simulink model "maddenlibrary"  (R2012b)
settings: Solver=ode45  StartTime=0.0  StopTime=10.0  RelTol=1e-3
values from neighbouring files (symbols this model uses):
  T = 95/2    (= 47.5)    [fluxrampdemodsim.m]
undefined symbols (not defined in the file or in its folder): A, FRA, FRT, pfb_coeff_gen_calc, RS, T2, V
undefined symbols (not defined in the file): SL, transtable
libraries: xbsIndex_r4 x10038, casper_library_misc x83, casper_library_delays x22, xps_library x19, simulink x3, maddogLibrary x1
(part 13 of 106)

== system maddenlibrary/FRD/PhaseUnwrap ==
  note: FixPosJump
  note: Fix Neg Jup
  note: Determine If Phase Jump
  note: Calculate if we have Phase Jump
      | by comparing derivative of phase wrt time
      | to pi and -pi.
  note: Perform Phase Unwrap by adding
      | 0 , 2pi or -2pi
  note: State 0 : Add 0 to phase
      | Sate 1: Add 2pi to phase
      | State 2: Add -2pi to phase
      | State 3: Error
  note: Phase Unwrap
  note: State Machine Next State
  note: Error Flag Output
  note: Phase Addend:
      | 0.0, 2pi or -2pi
  note: Calc. Unwrapped
      | Phase
  note: How the muxes work
      |
      | always @(posedge clk)
      | //NextStae Mux
      | switch State:
      | {
      | 	0: //add 0 to phase
      | 		switch {negjmp, posjmp}
      | 		{
      | 			0: state<=0; break;
      | 			1: state,=1;break
      | 			2:state <=2; break
      | 			3:state <=3;
      | 		}
      | 		break
      |
      | 	1: // add
  Phase : Inport
  Rst : Inport  Port=2
  vld_in : Inport  Port=3
  mag_in : Inport  Port=4
  AddSub : xbsIndex_r4/AddSub  mode=Addition  use_carryin=off  use_carryout=off  en=off  latency=1  precision=User Defined  arith_type="Signed  (2's comp)"  n_bits=16  bin_pt=13  quantization=Truncate  overflow=Wrap  dbl_ovrd=off  use_behavioral_HDL=off  hw_selection=Fabric  pipelined=off  block_type=addsub
  Concat : xbsIndex_r4/Concat  num_inputs=2  dbl_ovrd=off  block_type=concat
  Constant : xbsIndex_r4/Constant  const=0  gui_display_data_type=Fixed-point  arith_type=Signed (2's comp)  n_bits=16  bin_pt=13  preci_type=Single  exp_width=8  frac_width=24  explicit_period=on  period=1  equ=P=C  opselect=C  inp2=PCIN>>17  opr=+  inp1=P  carry=CIN  dbl_ovrd=off  block_type=constant
  Constant1 : xbsIndex_r4/Constant  const=2  gui_display_data_type=Fixed-point  arith_type=Signed (2's comp)  n_bits=16  bin_pt=13  preci_type=Single  exp_width=8  frac_width=24  explicit_period=on  period=1  equ=P=C  opselect=C  inp2=PCIN>>17  opr=+  inp1=P  carry=CIN  dbl_ovrd=off  block_type=constant
  Constant10 : xbsIndex_r4/Constant  const=0  gui_display_data_type=Fixed-point  arith_type=Unsigned  n_bits=2  bin_pt=0  preci_type=Single  exp_width=8  frac_width=24  explicit_period=on  period=1  equ=P=C  opselect=C  inp2=PCIN>>17  opr=+  inp1=P  carry=CIN  dbl_ovrd=off  block_type=constant
  Constant{8,11..13,15,17} (6 alike) : xbsIndex_r4/Constant  const=3  gui_display_data_type=Fixed-point  arith_type=Unsigned  n_bits=2  bin_pt=0  preci_type=Single  exp_width=8  frac_width=24  explicit_period=on  period=1  equ=P=C  opselect=C  inp2=PCIN>>17  opr=+  inp1=P  carry=CIN  dbl_ovrd=off  block_type=constant
  Constant14 : xbsIndex_r4/Constant  const=0  gui_display_data_type=Fixed-point  arith_type=Unsigned  n_bits=2  bin_pt=0  preci_type=Single  exp_width=8  frac_width=24  explicit_period=on  period=1  equ=P=C  opselect=C  inp2=PCIN>>17  opr=+  inp1=P  carry=CIN  dbl_ovrd=off  block_type=constant
  Constant16 : xbsIndex_r4/Constant  const=2  gui_display_data_type=Fixed-point  arith_type=Unsigned  n_bits=2  bin_pt=0  preci_type=Single  exp_width=8  frac_width=24  explicit_period=on  period=1  equ=P=C  opselect=C  inp2=PCIN>>17  opr=+  inp1=P  carry=CIN  dbl_ovrd=off  block_type=constant
  Constant18 : xbsIndex_r4/Constant  const=0  gui_display_data_type=Boolean  arith_type=Boolean  n_bits=2  bin_pt=0  preci_type=Single  exp_width=8  frac_width=24  explicit_period=on  period=1  equ=P=C  opselect=C  inp2=PCIN>>17  opr=+  inp1=P  carry=CIN  dbl_ovrd=off  block_type=constant
  Constant19 : xbsIndex_r4/Constant  const=1  gui_display_data_type=Boolean  arith_type=Boolean  n_bits=2  bin_pt=0  preci_type=Single  exp_width=8  frac_width=24  explicit_period=on  period=1  equ=P=C  opselect=C  inp2=PCIN>>17  opr=+  inp1=P  carry=CIN  dbl_ovrd=off  block_type=constant
  Constant2 : xbsIndex_r4/Constant  const=-2  gui_display_data_type=Fixed-point  arith_type=Signed (2's comp)  n_bits=16  bin_pt=13  preci_type=Single  exp_width=8  frac_width=24  explicit_period=on  period=1  equ=P=C  opselect=C  inp2=PCIN>>17  opr=+  inp1=P  carry=CIN  dbl_ovrd=off  block_type=constant
  Constant3 : xbsIndex_r4/Constant  const=-1  gui_display_data_type=Fixed-point  arith_type=Signed (2's comp)  n_bits=16  bin_pt=13  preci_type=Single  exp_width=8  frac_width=24  explicit_period=on  period=1  equ=P=C  opselect=C  inp2=PCIN>>17  opr=+  inp1=P  carry=CIN  dbl_ovrd=off  block_type=constant
  Constant4 : xbsIndex_r4/Constant  const=1.0  gui_display_data_type=Fixed-point  arith_type=Signed (2's comp)  n_bits=16  bin_pt=13  preci_type=Single  exp_width=8  frac_width=24  explicit_period=on  period=1  equ=P=C  opselect=C  inp2=PCIN>>17  opr=+  inp1=P  carry=CIN  dbl_ovrd=off  block_type=constant
  Constant5 : xbsIndex_r4/Constant  const=0  gui_display_data_type=Fixed-point  arith_type=Unsigned  n_bits=2  bin_pt=0  preci_type=Single  exp_width=8  frac_width=24  explicit_period=on  period=1  equ=P=C  opselect=C  inp2=PCIN>>17  opr=+  inp1=P  carry=CIN  dbl_ovrd=off  block_type=constant
  Constant6 : xbsIndex_r4/Constant  const=2  gui_display_data_type=Fixed-point  arith_type=Unsigned  n_bits=2  bin_pt=0  preci_type=Single  exp_width=8  frac_width=24  explicit_period=on  period=1  equ=P=C  opselect=C  inp2=PCIN>>17  opr=+  inp1=P  carry=CIN  dbl_ovrd=off  block_type=constant
  Constant7 : xbsIndex_r4/Constant  const=1  gui_display_data_type=Fixed-point  arith_type=Unsigned  n_bits=2  bin_pt=0  preci_type=Single  exp_width=8  frac_width=24  explicit_period=on  period=1  equ=P=C  opselect=C  inp2=PCIN>>17  opr=+  inp1=P  carry=CIN  dbl_ovrd=off  block_type=constant
  Constant9 : xbsIndex_r4/Constant  const=1  gui_display_data_type=Fixed-point  arith_type=Unsigned  n_bits=2  bin_pt=0  preci_type=Single  exp_width=8  frac_width=24  explicit_period=on  period=1  equ=P=C  opselect=C  inp2=PCIN>>17  opr=+  inp1=P  carry=CIN  dbl_ovrd=off  block_type=constant
  Delay : xbsIndex_r4/Delay  rst=off  infoeditControl=Selection of Reset will increase slice count due to use of real FFs and instead of SRLs  en=off  latency=1  dbl_ovrd=off  reg_retiming=off  block_type=delay
  Delay1 : xbsIndex_r4/Delay  rst=off  infoeditControl=Selection of Reset will increase slice count due to use of real FFs and instead of SRLs  en=off  latency=1  dbl_ovrd=off  reg_retiming=off  block_type=delay
  DiffPhase : xbsIndex_r4/AddSub  mode=Subtraction  use_carryin=off  use_carryout=off  en=off  latency=0  precision=Full  arith_type=Unsigned  n_bits=16  bin_pt=14  quantization=Truncate  overflow=Wrap  dbl_ovrd=off  use_behavioral_HDL=off  hw_selection=Fabric  pipelined=off  block_type=addsub
  ErrorOutput : xbsIndex_r4/Mux  inputs=4  en=off  latency=0  precision=Full  arith_type=Unsigned  n_bits=16  bin_pt=14  quantization=Truncate  overflow=Wrap  dbl_ovrd=off  block_type=mux
  NegativeJum : xbsIndex_r4/Relational  mode=a>b  en=off  latency=0  dbl_ovrd=off  block_type=relational
  NextState : xbsIndex_r4/Mux  inputs=4  en=off  latency=0  precision=Full  arith_type=Unsigned  n_bits=16  bin_pt=14  quantization=Truncate  overflow=Wrap  dbl_ovrd=off  block_type=mux
  PhaseAddend : xbsIndex_r4/Mux  inputs=4  en=off  latency=0  precision=Full  arith_type=Unsigned  n_bits=16  bin_pt=14  quantization=Truncate  overflow=Wrap  dbl_ovrd=off  block_type=mux
  PositiveJump : xbsIndex_r4/Relational  mode=a<b  en=off  latency=0  dbl_ovrd=off  block_type=relational
  State : xbsIndex_r4/Register  init=0  rst=on  en=on  dbl_ovrd=off  block_type=register
  StateNext0 : xbsIndex_r4/Mux  inputs=4  en=off  latency=0  precision=Full  arith_type=Unsigned  n_bits=16  bin_pt=14  quantization=Truncate  overflow=Wrap  dbl_ovrd=off  block_type=mux
  StateNext1 : xbsIndex_r4/Mux  inputs=4  en=off  latency=0  precision=Full  arith_type=Unsigned  n_bits=16  bin_pt=14  quantization=Truncate  overflow=Wrap  dbl_ovrd=off  block_type=mux
  StateNext2 : xbsIndex_r4/Mux  inputs=4  en=off  latency=0  precision=Full  arith_type=Unsigned  n_bits=16  bin_pt=14  quantization=Truncate  overflow=Wrap  dbl_ovrd=off  block_type=mux
  Wait_for_FSM : xbsIndex_r4/Delay  rst=off  infoeditControl=Selection of Reset will increase slice count due to use of real FFs and instead of SRLs  en=off  latency=1  dbl_ovrd=off  reg_retiming=off  block_type=delay
  Wait_for_FSM1 : xbsIndex_r4/Delay  rst=off  infoeditControl=Selection of Reset will increase slice count due to use of real FFs and instead of SRLs  en=off  latency=2  dbl_ovrd=off  reg_retiming=off  block_type=delay
  Wait_for_FSM2 : xbsIndex_r4/Delay  rst=off  infoeditControl=Selection of Reset will increase slice count due to use of real FFs and instead of SRLs  en=off  latency=2  dbl_ovrd=off  reg_retiming=off  block_type=delay
  UwrPhase : Outport
  Err : Outport  Port=2
  vld_out : Outport  Port=3
  mag_out : Outport  Port=4
  wires:
  Delay/1 -> DiffPhase/2
  Constant19/1 -> ErrorOutput/5
  NextState/1 -> State/1
  StateNext1/1 -> NextState/3
  Constant9/1 -> StateNext1/2
  PositiveJump/1 -> Concat/2
  Constant13/1 -> StateNext2/4
  Constant15/1 -> StateNext2/5
  DiffPhase/1 -> PositiveJump/1, NegativeJum/1
  State/1 -> ErrorOutput/1, PhaseAddend/1, NextState/1
  Constant10/1 -> StateNext1/4
  Constant11/1 -> StateNext1/3
  PhaseAddend/1 -> AddSub/2
  Constant2/1 -> PhaseAddend/4
  Concat/1 -> StateNext1/1, StateNext0/1, StateNext2/1
  Constant5/1 -> StateNext0/2
  ErrorOutput/1 -> Err/1
  Rst/1 -> State/2
  Constant17/1 -> NextState/5
  AddSub/1 -> UwrPhase/1
  Constant/1 -> PhaseAddend/5, PhaseAddend/2
  Phase/1 -> Delay/1, DiffPhase/1, Wait_for_FSM/1
  Constant4/1 -> NegativeJum/2
  StateNext0/1 -> NextState/2
  Constant16/1 -> StateNext2/2
  Constant14/1 -> StateNext2/3
  Constant12/1 -> StateNext1/5
  Wait_for_FSM/1 -> AddSub/1
  Constant8/1 -> StateNext0/5
  Constant7/1 -> StateNext0/3
  Constant18/1 -> ErrorOutput/4, ErrorOutput/3, ErrorOutput/2
  Constant6/1 -> StateNext0/4
  StateNext2/1 -> NextState/4
  NegativeJum/1 -> Concat/1
  Constant3/1 -> PositiveJump/2
  Constant1/1 -> PhaseAddend/3
  vld_in/1 -> Delay1/1, Wait_for_FSM1/1
  Wait_for_FSM1/1 -> vld_out/1
  Wait_for_FSM2/1 -> mag_out/1
  mag_in/1 -> Wait_for_FSM2/1
  Delay1/1 -> State/3

== system maddenlibrary/FRD/edge_detect1 ==
  in : Inport
  Delay : xbsIndex_r4/Delay  rst=off  infoeditControl=Selection of Reset will increase slice count due to use of real FFs and instead of SRLs  en=off  latency=1  dbl_ovrd=off  reg_retiming=off  block_type=delay
      settings: xl_area=[0, 0, 0, 0, 0, 0, 0]
  Inverter : xbsIndex_r4/Inverter  en=off  latency=0  dbl_ovrd=off  block_type=inv
      settings: xl_area=[0, 0, 0, 0, 0, 0, 0]
  edge_op : xbsIndex_r4/Logical  logical_function=NOR  inputs=2  en=off  latency=0  precision=Full  arith_type=Unsigned  n_bits=8  bin_pt=2  align_bp=on  dbl_ovrd=off  block_type=logical
      settings: xl_area=[0, 0, 0, 0, 0, 0, 0]
  out : Outport
  wires:
  Inverter/1 -> edge_op/1
  edge_op/1 -> out/1
  in/1 -> Inverter/1, Delay/1
  Delay/1 -> edge_op/2

== system maddenlibrary/FRD/flrampfsmoutst ==
  out_reg : Inport
  assert_reg : xbsIndex_r4/Assert  assert_type=on  type_source=Explicitly  gui_display_data_type=Fixed-point  arith_type=Unsigned  n_bits=5  bin_pt=0  preci_type=Single  exp_width=8  frac_width=24  assert_rate=off  rate_source=Explicitly  period=1  output_port=on  block_type=assert
  cast_gw : xbsIndex_r4/Convert  gui_display_data_type=Fixed-point  arith_type=Unsigned  n_bits=32  bin_pt=0  float_type=Single  exp_bits=8  fraction_bits=24  quantization=Truncate  overflow=Wrap  en=off  latency=0  dbl_ovrd=off  pipeline=off  block_type=convert
  io_delay : xbsIndex_r4/Delay  rst=off  infoeditControl=Selection of Reset will increase slice count due to use of real FFs and instead of SRLs  en=off  latency=0  dbl_ovrd=off  reg_retiming=on  block_type=delay
  maddenlibrary_FRD_flrampfsmoutst_user_data_in : xbsIndex_r4/Gateway Out  inherit_from_input=off  hdl_port=on  timing_constraint=None  locs_specified=off  LOCs={}  UseAsDAC=off  DACChannel='1'  block_type=gatewayout
  reint1 : xbsIndex_r4/Reinterpret  force_arith_type=on  arith_type=Unsigned  force_bin_pt=on  bin_pt=0  block_type=reinterpret
  sim_out : Outport
  wires:
  io_delay/1 -> cast_gw/1
  cast_gw/1 -> maddenlibrary_FRD_flrampfsmoutst_user_data_in/1
  maddenlibrary_FRD_flrampfsmoutst_user_data_in/1 -> sim_out/1
  out_reg/1 -> assert_reg/1
  assert_reg/1 -> reint1/1
  reint1/1 -> io_delay/1

== system maddenlibrary/FRD/flrampfsmst ==
  out_reg : Inport
  assert_reg : xbsIndex_r4/Assert  assert_type=on  type_source=Explicitly  gui_display_data_type=Fixed-point  arith_type=Unsigned  n_bits=4  bin_pt=0  preci_type=Single  exp_width=8  frac_width=24  assert_rate=off  rate_source=Explicitly  period=1  output_port=on  block_type=assert
  cast_gw : xbsIndex_r4/Convert  gui_display_data_type=Fixed-point  arith_type=Unsigned  n_bits=32  bin_pt=0  float_type=Single  exp_bits=8  fraction_bits=24  quantization=Truncate  overflow=Wrap  en=off  latency=0  dbl_ovrd=off  pipeline=off  block_type=convert
  io_delay : xbsIndex_r4/Delay  rst=off  infoeditControl=Selection of Reset will increase slice count due to use of real FFs and instead of SRLs  en=off  latency=0  dbl_ovrd=off  reg_retiming=on  block_type=delay
  maddenlibrary_FRD_flrampfsmst_user_data_in : xbsIndex_r4/Gateway Out  inherit_from_input=off  hdl_port=on  timing_constraint=None  locs_specified=off  LOCs={}  UseAsDAC=off  DACChannel='1'  block_type=gatewayout
  reint1 : xbsIndex_r4/Reinterpret  force_arith_type=on  arith_type=Unsigned  force_bin_pt=on  bin_pt=0  block_type=reinterpret
  sim_out : Outport
  wires:
  io_delay/1 -> cast_gw/1
  cast_gw/1 -> maddenlibrary_FRD_flrampfsmst_user_data_in/1
  maddenlibrary_FRD_flrampfsmst_user_data_in/1 -> sim_out/1
  out_reg/1 -> assert_reg/1
  assert_reg/1 -> reint1/1
  reint1/1 -> io_delay/1

== system maddenlibrary/FRD/trIQ ==
  note: Translation in IQ Plane
  Q : Inport
  I : Inport  Port=2
  vld_in : Inport  Port=3
  chan : Inport  Port=4
  Constant : xbsIndex_r4/Constant  const=0  gui_display_data_type=Fixed-point  arith_type=Unsigned  n_bits=32  bin_pt=0  preci_type=Single  exp_width=8  frac_width=24  explicit_period=on  period=1  equ=P=C  opselect=C  inp2=PCIN>>17  opr=+  inp1=P  carry=CIN  dbl_ovrd=off  block_type=constant
  Constant1 : xbsIndex_r4/Constant  const=0  gui_display_data_type=Boolean  arith_type=Boolean  n_bits=16  bin_pt=14  preci_type=Single  exp_width=8  frac_width=24  explicit_period=on  period=1  equ=P=C  opselect=C  inp2=PCIN>>17  opr=+  inp1=P  carry=CIN  dbl_ovrd=off  block_type=constant
  Convert : xbsIndex_r4/Convert  gui_display_data_type=Fixed-point  arith_type=Unsigned  n_bits=10  bin_pt=0  float_type=Single  exp_bits=8  fraction_bits=24  quantization=Truncate  overflow=Wrap  en=off  latency=0  dbl_ovrd=off  pipeline=off  block_type=convert
  Delay : xbsIndex_r4/Delay  rst=off  infoeditControl=Selection of Reset will increase slice count due to use of real FFs and instead of SRLs  en=off  latency=1  dbl_ovrd=off  reg_retiming=off  block_type=delay
  LSW : xbsIndex_r4/Slice  nbits=16  boolean_output=off  mode=Lower Bit Location + Width  bit1=0  base1=MSB of Input  bit0=0  base0=LSB of Input  dbl_ovrd=off  block_type=slice
  MSW : xbsIndex_r4/Slice  nbits=16  boolean_output=off  mode=Upper Bit Location + Width  bit1=0  base1=MSB of Input  bit0=0  base0=LSB of Input  dbl_ovrd=off  block_type=slice
  int16_14_ : xbsIndex_r4/Reinterpret  force_arith_type=on  arith_type="Signed  (2's comp)"  force_bin_pt=on  bin_pt=14  block_type=reinterpret
  int16_14_1 : xbsIndex_r4/Reinterpret  force_arith_type=on  arith_type="Signed  (2's comp)"  force_bin_pt=on  bin_pt=14  block_type=reinterpret
  tr : Subsystem  Tag=xps:bram  AncestorBlock=xps_library/Shared BRAM  mask{arith_type=Unsigned, addr_width=10, data_width=32, reg_prim_output=off, reg_core_output=off, optimization=Minimum_Area, data_bin_pt=0, init_vals=transtable, sample_rate=1}
      mask prompts: arith_type "Output Data Type"; addr_width "Address width"; data_width "Data Width"; reg_prim_output "Register Primitive Output"; reg_core_output "Register Core Output"; data_bin_pt "Data Binary Point"; init_vals "Initial values (simulation only)"; sample_rate "Sample rate"
      mask init:
      | shared_bram_mask;
      mask TypeOptions arith_type: Unsigned | Signed  (2's comp)
      mask TypeOptions data_width: 8 | 16 | 32 | 64 | 128
      mask TypeOptions optimization: Minimum_Area | Low_Power
  trotimag : xbsIndex_r4/AddSub  mode=Addition  use_carryin=off  use_carryout=off  en=off  latency=1  precision=User Defined  arith_type="Signed  (2's comp)"  n_bits=16  bin_pt=14  quantization=Truncate  overflow=Wrap  dbl_ovrd=off  use_behavioral_HDL=off  hw_selection=Fabric  pipelined=off  block_type=addsub
  trotreal : xbsIndex_r4/AddSub  mode=Addition  use_carryin=off  use_carryout=off  en=off  latency=1  precision=User Defined  arith_type="Signed  (2's comp)"  n_bits=16  bin_pt=14  quantization=Truncate  overflow=Wrap  dbl_ovrd=off  use_behavioral_HDL=off  hw_selection=Fabric  pipelined=off  block_type=addsub
  Qt : Outport
  It : Outport  Port=2
  vld_out : Outport  Port=3
  wires:
  Q/1 -> trotimag/2
  int16_14_/1 -> trotimag/1
  I/1 -> trotreal/1
  int16_14_1/1 -> trotreal/2
  trotreal/1 -> It/1
  trotimag/1 -> Qt/1
  Delay/1 -> vld_out/1
  vld_in/1 -> Delay/1
  Convert/1 -> tr/1(addr)
  chan/1 -> Convert/1
  Constant1/1 -> tr/3(we)
  Constant/1 -> tr/2(data_in)
  tr/1(data_out) -> MSW/1, LSW/1
  LSW/1 -> int16_14_/1
  MSW/1 -> int16_14_1/1

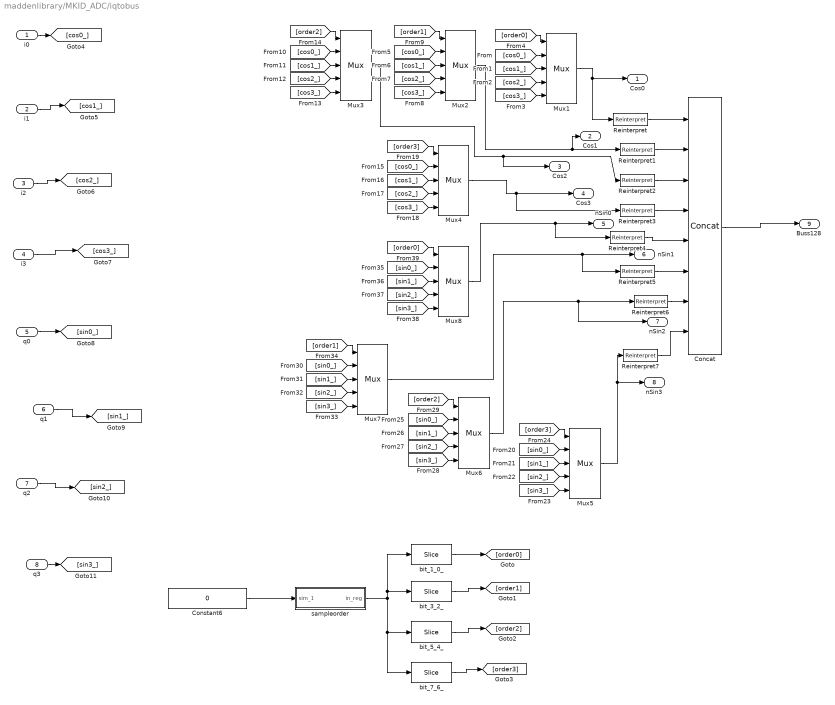
== system maddenlibrary/MKID_ADC/iqtobus ==
  i0 : Inport
  i1 : Inport  Port=2
  i2 : Inport  Port=3
  i3 : Inport  Port=4
  q0 : Inport  Port=5
  q1 : Inport  Port=6
  q2 : Inport  Port=7
  q3 : Inport  Port=8
  Concat : xbsIndex_r4/Concat  num_inputs=8  dbl_ovrd=off  block_type=concat
  Constant6 : Constant  Value=0
  Mux{1..8} (8 alike) : xbsIndex_r4/Mux  inputs=4  en=off  latency=1  precision=Full  arith_type=Unsigned  n_bits=16  bin_pt=14  quantization=Truncate  overflow=Wrap  dbl_ovrd=off  block_type=mux
  Reinterpret{,1..7} (8 alike) : xbsIndex_r4/Reinterpret  force_arith_type=on  arith_type=Unsigned  force_bin_pt=on  bin_pt=0  block_type=reinterpret
  bit_1_0_ : xbsIndex_r4/Slice  nbits=2  boolean_output=off  mode=Lower Bit Location + Width  bit1=0  base1=MSB of Input  bit0=0  base0=LSB of Input  dbl_ovrd=off  block_type=slice
  bit_3_2_ : xbsIndex_r4/Slice  nbits=2  boolean_output=off  mode=Lower Bit Location + Width  bit1=0  base1=MSB of Input  bit0=2  base0=LSB of Input  dbl_ovrd=off  block_type=slice
  bit_5_4_ : xbsIndex_r4/Slice  nbits=2  boolean_output=off  mode=Lower Bit Location + Width  bit1=0  base1=MSB of Input  bit0=4  base0=LSB of Input  dbl_ovrd=off  block_type=slice
  bit_7_6_ : xbsIndex_r4/Slice  nbits=2  boolean_output=off  mode=Lower Bit Location + Width  bit1=0  base1=MSB of Input  bit0=6  base0=LSB of Input  dbl_ovrd=off  block_type=slice
  sampleorder : Subsystem  Tag=xps:sw_reg  AncestorBlock=xps_library/software register  mask(swreg){mode=one value, io_dir=From Processor, io_delay=0, sample_period=1, names=reg, bitwidths=32, arith_types=0, bin_pts=0, sim_port=on, show_format=off}
      mask prompts: io_dir "I/O direction"; io_delay "I/O delay"; sample_period "Sample period"; names "Name:"; bitwidths "Bitwidth:"; arith_types "Type (ufix=0, fix=1, bool=2):"; bin_pts "Binary pt:"; sim_port "Provide sim input/output?"; show_format "Print format string?"
      mask init:
      | swreg_init(gcb)
      settings: AttributesFormatString=1input
      mask TypeOptions mode: one value | fields of equal size | fields of arbitrary size
      mask Callback mode: swreg_cb(gcb);
      mask TypeOptions io_dir: To Processor | From Processor
      mask Callback io_dir:
      | mask_enables = get_param(gcb, 'MaskEnables');
      | mask_names = get_param(gcb, 'MaskNames');
      | if strcmp(get_param(gcb, 'io_dir'), 'To Processor'),
      |     mask_enables{ismember(mask_names, 'sample_period')} = 'off';
      | else
      |     mask_enables{ismember(mask_names, 'sample_period')} = 'on';
      | end
      | set_param(gcb, 'MaskEnables', mask_enables);
      mask Callback bitwidths:
      | swreg_maskcheck(gcb);
      | % blk = gcb;
      | % mode = get_param(blk, 'mode');
      | % current_widths = eval(get_param(blk, 'bitwidths'));
      | % if (strcmp(mode, 'one value') || strcmp(mode, 'fields of equal size')) && (length(current_widths) > 1),
      | %     error('Only one width may be specified for this mode.');
      | % elseif strcmp(mode, 'fields of arbitrary size')
      | %     current_names = textscan(strtrim(strrep(strrep(get_param(blk, 'names'), ']', ''), '[', '')), '%s');
      | %     current_names = current_names{1};
      | %     numios = length(current_names);
      | %     if length(current_widths) ~= numios,
      | %         error('%d field names specified, but %d widths?', numios, length(current_widths));
      | %     end
      | % end
      | % total_width = 0;
      | % for ctr = 1 : length(current_widths),
      | %     total_width = total_width + current_widths(ctr);
      | % end
      | % if total_width > 32,
      | %     error('Total width must be 32 or less, set to %d.', total_width);
      | % end
      mask Callback arith_types:
      | [numios, ~, ~, ~, current_types] = swreg_maskcheck(gcb);
      | % blk = gcb;
      | % mode = get_param(blk, 'mode');
      | % current_types = eval(get_param(blk, 'arith_types'));
      | % numios = length(current_types);
      | % if (strcmp(mode, 'one value') || strcmp(mode, 'fields of equal size')) && (length(current_types) > 1),
      | %     error('Only one type may be specified for this mode.');
      | % elseif strcmp(mode, 'fields of arbitrary size')
      | %     current_names = textscan(strtrim(strrep(strrep(get_param(blk, 'names'), ']', ''), '[', '')), '%s');
      | %     current_names = current_names{1};
      | %     numios = length(current_names);
      | %     if length(current_types) ~= numios,
      | %         error('%d field names specified, but %d types?', numios, length(current_types));
      | %     end
      | % end
      | problem = 0;
      | for ctr = 1 : numios,
      |     t = current_types(ctr);
      |     if (t < 0) || (t > 2),
      |         problem = t;
      |         ctr = numios + 1;
      |     end
      | end
      | if problem ~= 0,
      |     error('Type cannot be %i, must be 0, 1 or 2.', problem);
      | end
      mask Callback bin_pts:
      | swreg_maskcheck(gcb);
      | % blk = gcb;
      | % mode = get_param(blk, 'mode');
      | % current_bins = eval(get_param(blk, 'bin_pts'));
      | % if (strcmp(mode, 'one value') || strcmp(mode, 'fields of equal size')) && (length(current_bins) > 1),
      | %     error('Only one binary pt may be specified for this mode.');
      | % elseif strcmp(mode, 'fields of arbitrary size')
      | %     current_names = textscan(strtrim(strrep(strrep(get_param(blk, 'names'), ']', ''), '[', '')), '%s');
      | %     current_names = current_names{1};
      | %     numios = length(current_names);
      | %     if length(current_bins) ~= numios,
      | %         error('%d field names specified, but %d binary pts?', numios, length(current_bins));
      | %     end
      | % end
  Cos0 : Outport
  Cos1 : Outport  Port=2
  Cos2 : Outport  Port=3
  Cos3 : Outport  Port=4
  nSin0 : Outport  Port=5
  nSin1 : Outport  Port=6
  nSin2 : Outport  Port=7
  nSin3 : Outport  Port=8
  Buss128 : Outport  Port=9
  wires:
  Reinterpret4/1 -> Concat/5
  [cos2_] -> Mux2/4
  [sin0_] -> Mux5/2
  [cos0_] -> Mux4/2
  Constant6/1 -> sampleorder/1(sim_1)
  [sin1_] -> Mux5/3
  Reinterpret1/1 -> Concat/2
  Reinterpret/1 -> Concat/1
  [cos2_] -> Mux1/4
  bit_3_2_/1 -> [order1]
  Reinterpret3/1 -> Concat/4
  [cos0_] -> Mux3/2
  [cos1_] -> Mux4/3
  bit_7_6_/1 -> [order3]
  [cos0_] -> Mux1/2
  Mux7/1 -> nSin1/1, Reinterpret5/1
  Mux1/1 -> Reinterpret/1, Cos0/1
  Mux8/1 -> nSin0/1, Reinterpret4/1
  Reinterpret5/1 -> Concat/6
  [sin2_] -> Mux5/4
  Mux4/1 -> Cos3/1, Reinterpret3/1
  [cos1_] -> Mux1/3
  Reinterpret6/1 -> Concat/7
  [order3] -> Mux5/1
  Concat/1 -> Buss128/1
  [cos3_] -> Mux1/5
  Mux2/1 -> Cos1/1, Reinterpret1/1
  [cos2_] -> Mux4/4
  sampleorder/1(in_reg) -> bit_7_6_/1, bit_5_4_/1, bit_3_2_/1, bit_1_0_/1
  Mux5/1 -> nSin3/1, Reinterpret7/1
  [sin2_] -> Mux8/4
  [order1] -> Mux7/1
  [cos3_] -> Mux3/5
  [order1] -> Mux2/1
  [order2] -> Mux6/1
  i0/1 -> [cos0_]
  Mux6/1 -> nSin2/1, Reinterpret6/1
  [cos2_] -> Mux3/4
  [sin0_] -> Mux7/2
  [cos0_] -> Mux2/2
  [sin3_] -> Mux7/5
  [sin2_] -> Mux7/4
  [cos1_] -> Mux3/3
  [sin0_] -> Mux8/2
  [order0] -> Mux8/1
  [sin3_] -> Mux5/5
  bit_1_0_/1 -> [order0]
  [cos3_] -> Mux4/5
  [sin1_] -> Mux7/3
  [cos1_] -> Mux2/3
  [sin1_] -> Mux8/3
  [order3] -> Mux4/1
  [sin1_] -> Mux6/3
  Reinterpret7/1 -> Concat/8
  q3/1 -> [sin3_]
  [sin3_] -> Mux6/5
  Mux3/1 -> Cos2/1, Reinterpret2/1
  bit_5_4_/1 -> [order2]
  [sin3_] -> Mux8/5
  [sin2_] -> Mux6/4
  Reinterpret2/1 -> Concat/3
  [cos3_] -> Mux2/5
  [order0] -> Mux1/1
  [order2] -> Mux3/1
  [sin0_] -> Mux6/2
  q2/1 -> [sin2_]
  q1/1 -> [sin1_]
  q0/1 -> [sin0_]
  i3/1 -> [cos3_]
  i1/1 -> [cos1_]
  i2/1 -> [cos2_]

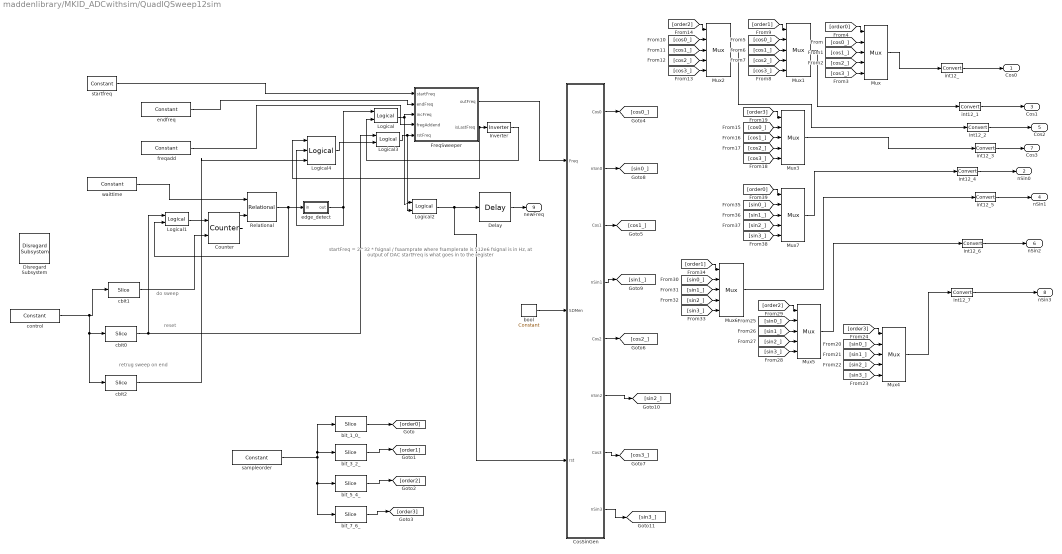
== system maddenlibrary/MKID_ADCwithsim/QuadIQSweep12sim ==
  note: retrug sweep on end
  note: do sweep
  note: reset
  note: startFreq = 2^32 * fsignal / fsaamprate
      | where fsamplerate is 512e6
      | fsignal is in Hz, at output of DAC
      | startFreq is what goes in to the register
  CosSinGen : Subsystem
  Counter : xbsIndex_r4/Counter  cnt_type=Free Running  cnt_to=Inf  operation=Up  start_count=0  cnt_by_val=1  arith_type=Unsigned  n_bits=32  bin_pt=0  load_pin=off  rst=on  en=on  explicit_period=on  period=1  dbl_ovrd=off  use_behavioral_HDL=off  implementation=Fabric  block_type=counter
  Delay : xbsIndex_r4/Delay  rst=off  infoeditControl=Selection of Reset will increase slice count due to use of real FFs and instead of SRLs  en=off  latency=4  dbl_ovrd=off  reg_retiming=off  block_type=delay
  Disregard Subsystem : xbsIndex_r4/Disregard Subsystem  Tag=discardX  block_type=disregard
  FreqSweeper : Subsystem
  Inverter : xbsIndex_r4/Inverter  en=off  latency=0  dbl_ovrd=off  block_type=inv
  Logical : xbsIndex_r4/Logical  logical_function=AND  inputs=2  en=off  latency=0  precision=Full  arith_type=Unsigned  n_bits=16  bin_pt=0  align_bp=on  dbl_ovrd=off  block_type=logical
  Logical1 : xbsIndex_r4/Logical  logical_function=OR  inputs=2  en=off  latency=0  precision=Full  arith_type=Unsigned  n_bits=16  bin_pt=0  align_bp=on  dbl_ovrd=off  block_type=logical
  Logical2 : xbsIndex_r4/Logical  logical_function=OR  inputs=2  en=off  latency=0  precision=Full  arith_type=Unsigned  n_bits=16  bin_pt=0  align_bp=on  dbl_ovrd=off  block_type=logical
  Logical3 : xbsIndex_r4/Logical  logical_function=OR  inputs=2  en=off  latency=0  precision=Full  arith_type=Unsigned  n_bits=16  bin_pt=0  align_bp=on  dbl_ovrd=off  block_type=logical
  Logical4 : xbsIndex_r4/Logical  logical_function=AND  inputs=3  en=off  latency=0  precision=Full  arith_type=Unsigned  n_bits=16  bin_pt=0  align_bp=on  dbl_ovrd=off  block_type=logical
  Mux{,1..7} (8 alike) : xbsIndex_r4/Mux  inputs=4  en=off  latency=1  precision=Full  arith_type=Unsigned  n_bits=16  bin_pt=14  quantization=Truncate  overflow=Wrap  dbl_ovrd=off  block_type=mux
  Relational : xbsIndex_r4/Relational  mode=a=b  en=off  latency=0  dbl_ovrd=off  block_type=relational
  bit_1_0_ : xbsIndex_r4/Slice  nbits=2  boolean_output=off  mode=Lower Bit Location + Width  bit1=0  base1=MSB of Input  bit0=0  base0=LSB of Input  dbl_ovrd=off  block_type=slice
  bit_3_2_ : xbsIndex_r4/Slice  nbits=2  boolean_output=off  mode=Lower Bit Location + Width  bit1=0  base1=MSB of Input  bit0=2  base0=LSB of Input  dbl_ovrd=off  block_type=slice
  bit_5_4_ : xbsIndex_r4/Slice  nbits=2  boolean_output=off  mode=Lower Bit Location + Width  bit1=0  base1=MSB of Input  bit0=4  base0=LSB of Input  dbl_ovrd=off  block_type=slice
  bit_7_6_ : xbsIndex_r4/Slice  nbits=2  boolean_output=off  mode=Lower Bit Location + Width  bit1=0  base1=MSB of Input  bit0=6  base0=LSB of Input  dbl_ovrd=off  block_type=slice
  bool : xbsIndex_r4/Constant  const=1  gui_display_data_type=Boolean  arith_type=Boolean  n_bits=16  bin_pt=14  preci_type=Single  exp_width=8  frac_width=24  explicit_period=on  period=1  equ=P=C  opselect=C  inp2=PCIN>>17  opr=+  inp1=P  carry=CIN  dbl_ovrd=off  block_type=constant
  cbit0 : xbsIndex_r4/Slice  nbits=1  boolean_output=on  mode=Lower Bit Location + Width  bit1=0  base1=MSB of Input  bit0=0  base0=LSB of Input  dbl_ovrd=off  block_type=slice
  cbit1 : xbsIndex_r4/Slice  nbits=1  boolean_output=on  mode=Lower Bit Location + Width  bit1=0  base1=MSB of Input  bit0=1  base0=LSB of Input  dbl_ovrd=off  block_type=slice
  cbit2 : xbsIndex_r4/Slice  nbits=1  boolean_output=on  mode=Lower Bit Location + Width  bit1=0  base1=MSB of Input  bit0=2  base0=LSB of Input  dbl_ovrd=off  block_type=slice
  control : xbsIndex_r4/Constant  const=6  gui_display_data_type=Fixed-point  arith_type=Unsigned  n_bits=32  bin_pt=0  preci_type=Single  exp_width=8  frac_width=24  explicit_period=on  period=1  equ=P=C  opselect=C  inp2=PCIN>>17  opr=+  inp1=P  carry=CIN  dbl_ovrd=off  block_type=constant
  edge_detect : Subsystem  AncestorBlock=casper_library_misc/edge_detect  mask(edge_detect){edge=Rising, polarity=Active High, x_in=[0 0.08 0.08 0.16 0.16 0.24 0.24 0.32 0.32 0.4], y_in=[-1 -1  1  1  1  1  1  1  1  1], x_out=[0.6 0.68 0.68 0.76 0.76 0.84 0.84 0.92 0.92 1], y_out=[-1 -1  1  1 -1 -1 -1 -1 -1 -1]}
      mask prompts: edge "Edge Type"; polarity "Output Polarity"; x_in "Input X Positions"; y_in "Input Y Positions"; x_out "Output X Positions"; y_out "Output Y Positions"
      mask help: Output is active for one-cycle after each edge of the specified type (i.e. rising, falling or both).
      mask init: same as maddenlibrary/DRAM_LUT/edge_detect
      settings: AttributesFormatString=|
      | rising edges
      | active high
      mask Help: Output is active for one-cycle after each edge of the specified type (i.e. rising, falling, or both).  Latency is zero.
      mask TypeOptions edge: Rising | Falling | Both
      mask TypeOptions polarity: Active High | Active Low
      mask Display:
      | plot(x_in_num,0.5+y_in_num*0.2);
      | plot(x_out_num,0.5+y_out_num*0.2);
  endfreq : xbsIndex_r4/Constant  const=238860800  gui_display_data_type=Fixed-point  arith_type=Unsigned  n_bits=32  bin_pt=0  preci_type=Single  exp_width=8  frac_width=24  explicit_period=on  period=1  equ=P=C  opselect=C  inp2=PCIN>>17  opr=+  inp1=P  carry=CIN  dbl_ovrd=off  block_type=constant
  freqadd : xbsIndex_r4/Constant  const=2388608  gui_display_data_type=Fixed-point  arith_type=Unsigned  n_bits=32  bin_pt=0  preci_type=Single  exp_width=8  frac_width=24  explicit_period=on  period=1  equ=P=C  opselect=C  inp2=PCIN>>17  opr=+  inp1=P  carry=CIN  dbl_ovrd=off  block_type=constant
  int12_{,1..7} (8 alike) : xbsIndex_r4/Convert  gui_display_data_type=Fixed-point  arith_type="Signed  (2's comp)"  n_bits=12  bin_pt=11  float_type=Single  exp_bits=8  fraction_bits=24  quantization=Truncate  overflow=Wrap  en=off  latency=0  dbl_ovrd=off  pipeline=off  block_type=convert
  sampleorder : xbsIndex_r4/Constant  const="0  + 1*4+  2*16 +  3*128"  gui_display_data_type=Fixed-point  arith_type=Unsigned  n_bits=32  bin_pt=0  preci_type=Single  exp_width=8  frac_width=24  explicit_period=on  period=1  equ=P=C  opselect=C  inp2=PCIN>>17  opr=+  inp1=P  carry=CIN  dbl_ovrd=off  block_type=constant
  startfreq : xbsIndex_r4/Constant  const=23886080  gui_display_data_type=Fixed-point  arith_type=Unsigned  n_bits=32  bin_pt=0  preci_type=Single  exp_width=8  frac_width=24  explicit_period=on  period=1  equ=P=C  opselect=C  inp2=PCIN>>17  opr=+  inp1=P  carry=CIN  dbl_ovrd=off  block_type=constant
  waittime : xbsIndex_r4/Constant  const=1024  gui_display_data_type=Fixed-point  arith_type=Unsigned  n_bits=32  bin_pt=0  preci_type=Single  exp_width=8  frac_width=24  explicit_period=on  period=1  equ=P=C  opselect=C  inp2=PCIN>>17  opr=+  inp1=P  carry=CIN  dbl_ovrd=off  block_type=constant
  Cos0 : Outport
  nSin0 : Outport  Port=2
  Cos1 : Outport  Port=3
  nSin1 : Outport  Port=4
  Cos2 : Outport  Port=5
  nSin2 : Outport  Port=6
  Cos3 : Outport  Port=7
  nSin3 : Outport  Port=8
  newFreq : Outport  Port=9
  wires:
  Relational/1 -> Logical1/2, edge_detect/1(in)
  Mux2/1 -> int12_2/1
  Counter/1 -> Relational/2
  edge_detect/1(out) -> Logical/1, Logical4/2
  cbit0/1 -> Logical1/1, Logical3/1
  freqadd/1 -> FreqSweeper/4(fregAddend)
  FreqSweeper/2(isLastFreq) -> Logical4/1, Inverter/1
  endfreq/1 -> FreqSweeper/2(endFreq)
  waittime/1 -> Relational/1
  Logical/1 -> Logical2/1, FreqSweeper/3(incFreq)
  cbit1/1 -> Counter/2
  FreqSweeper/1(outFreq) -> CosSinGen/1(Freq)
  bool/1 -> CosSinGen/2(SDMen)
  Logical1/1 -> Counter/1
  control/1 -> cbit2/1, cbit0/1, cbit1/1
  Inverter/1 -> Logical/2
  Mux/1 -> int12_/1
  Mux1/1 -> int12_1/1
  startfreq/1 -> FreqSweeper/1(startFreq)
  Delay/1 -> newFreq/1
  Logical2/1 -> Delay/1, CosSinGen/3(rst)
  Logical3/1 -> Logical2/2, FreqSweeper/5(rstFreq)
  cbit2/1 -> Logical4/3
  Logical4/1 -> Logical3/2
  sampleorder/1 -> bit_7_6_/1, bit_5_4_/1, bit_3_2_/1, bit_1_0_/1
  bit_1_0_/1 -> [order0]
  bit_3_2_/1 -> [order1]
  bit_5_4_/1 -> [order2]
  bit_7_6_/1 -> [order3]
  CosSinGen/1(Cos0) -> [cos0_]
  CosSinGen/3(Cos1) -> [cos1_]
  CosSinGen/5(Cos2) -> [cos2_]
  CosSinGen/7(Cos3) -> [cos3_]
  [cos0_] -> Mux/2
  [cos1_] -> Mux/3
  [cos2_] -> Mux/4
  [cos3_] -> Mux/5
  [order0] -> Mux/1
  [cos0_] -> Mux1/2
  [cos1_] -> Mux1/3
  [cos2_] -> Mux1/4
  [cos3_] -> Mux1/5
  [order1] -> Mux1/1
  [cos0_] -> Mux2/2
  [cos1_] -> Mux2/3
  [cos2_] -> Mux2/4
  [cos3_] -> Mux2/5
  [order2] -> Mux2/1
  [cos0_] -> Mux3/2
  [cos1_] -> Mux3/3
  [cos2_] -> Mux3/4
  [cos3_] -> Mux3/5
  [order3] -> Mux3/1
  Mux3/1 -> int12_3/1
  CosSinGen/8(nSin3) -> [sin3_]
  CosSinGen/6(nSin2) -> [sin2_]
  CosSinGen/4(nSin1) -> [sin1_]
  [sin0_] -> Mux4/2
  [sin1_] -> Mux4/3
  [sin2_] -> Mux4/4
  [sin3_] -> Mux4/5
  [order3] -> Mux4/1
  Mux4/1 -> int12_7/1
  [sin0_] -> Mux5/2
  [sin1_] -> Mux5/3
  [sin2_] -> Mux5/4
  [sin3_] -> Mux5/5
  [order2] -> Mux5/1
  [sin0_] -> Mux6/2
  [sin1_] -> Mux6/3
  [sin2_] -> Mux6/4
  [sin3_] -> Mux6/5
  [order1] -> Mux6/1
  [sin0_] -> Mux7/2
  [sin1_] -> Mux7/3
  [sin2_] -> Mux7/4
  [sin3_] -> Mux7/5
  [order0] -> Mux7/1
  Mux7/1 -> int12_4/1
  Mux6/1 -> int12_5/1
  Mux5/1 -> int12_6/1
  CosSinGen/2(nSin0) -> [sin0_]
  int12_1/1 -> Cos1/1
  int12_/1 -> Cos0/1
  int12_2/1 -> Cos2/1
  int12_3/1 -> Cos3/1
  int12_4/1 -> nSin0/1
  int12_5/1 -> nSin1/1
  int12_6/1 -> nSin2/1
  int12_7/1 -> nSin3/1

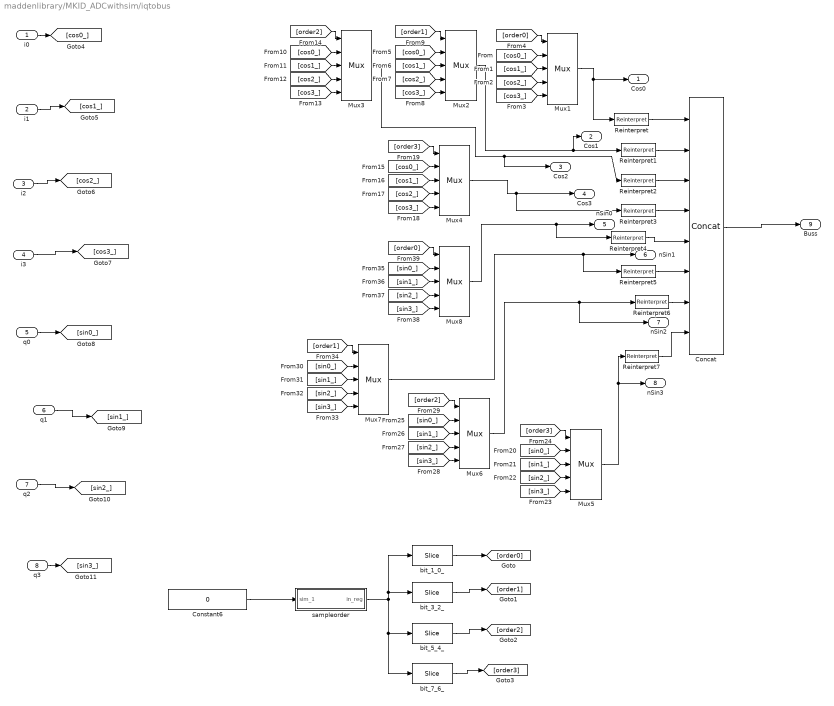
== system maddenlibrary/MKID_ADCwithsim/iqtobus ==
  i0 : Inport
  i1 : Inport  Port=2
  i2 : Inport  Port=3
  i3 : Inport  Port=4
  q0 : Inport  Port=5
  q1 : Inport  Port=6
  q2 : Inport  Port=7
  q3 : Inport  Port=8
  Concat : xbsIndex_r4/Concat  num_inputs=8  dbl_ovrd=off  block_type=concat
  Constant6 : Constant  Value=0
  Mux{1..8} (8 alike) : xbsIndex_r4/Mux  inputs=4  en=off  latency=1  precision=Full  arith_type=Unsigned  n_bits=16  bin_pt=14  quantization=Truncate  overflow=Wrap  dbl_ovrd=off  block_type=mux
  Reinterpret{,1..7} (8 alike) : xbsIndex_r4/Reinterpret  force_arith_type=on  arith_type=Unsigned  force_bin_pt=on  bin_pt=0  block_type=reinterpret
  bit_1_0_ : xbsIndex_r4/Slice  nbits=2  boolean_output=off  mode=Lower Bit Location + Width  bit1=0  base1=MSB of Input  bit0=0  base0=LSB of Input  dbl_ovrd=off  block_type=slice
  bit_3_2_ : xbsIndex_r4/Slice  nbits=2  boolean_output=off  mode=Lower Bit Location + Width  bit1=0  base1=MSB of Input  bit0=2  base0=LSB of Input  dbl_ovrd=off  block_type=slice
  bit_5_4_ : xbsIndex_r4/Slice  nbits=2  boolean_output=off  mode=Lower Bit Location + Width  bit1=0  base1=MSB of Input  bit0=4  base0=LSB of Input  dbl_ovrd=off  block_type=slice
  bit_7_6_ : xbsIndex_r4/Slice  nbits=2  boolean_output=off  mode=Lower Bit Location + Width  bit1=0  base1=MSB of Input  bit0=6  base0=LSB of Input  dbl_ovrd=off  block_type=slice
  sampleorder : Subsystem  Tag=xps:sw_reg  AncestorBlock=xps_library/software register  mask(swreg){mode=one value, io_dir=From Processor, io_delay=0, sample_period=1, names=reg, bitwidths=32, arith_types=0, bin_pts=0, sim_port=on, show_format=off}
      mask prompts: io_dir "I/O direction"; io_delay "I/O delay"; sample_period "Sample period"; names "Name:"; bitwidths "Bitwidth:"; arith_types "Type (ufix=0, fix=1, bool=2):"; bin_pts "Binary pt:"; sim_port "Provide sim input/output?"; show_format "Print format string?"
      mask init:
      | swreg_init(gcb)
      settings: AttributesFormatString=1input
      mask TypeOptions mode: one value | fields of equal size | fields of arbitrary size
      mask Callback mode: swreg_cb(gcb);
      mask TypeOptions io_dir: To Processor | From Processor
      mask Callback io_dir:
      | mask_enables = get_param(gcb, 'MaskEnables');
      | mask_names = get_param(gcb, 'MaskNames');
      | if strcmp(get_param(gcb, 'io_dir'), 'To Processor'),
      |     mask_enables{ismember(mask_names, 'sample_period')} = 'off';
      | else
      |     mask_enables{ismember(mask_names, 'sample_period')} = 'on';
      | end
      | set_param(gcb, 'MaskEnables', mask_enables);
      mask Callback bitwidths:
      | swreg_maskcheck(gcb);
      | % blk = gcb;
      | % mode = get_param(blk, 'mode');
      | % current_widths = eval(get_param(blk, 'bitwidths'));
      | % if (strcmp(mode, 'one value') || strcmp(mode, 'fields of equal size')) && (length(current_widths) > 1),
      | %     error('Only one width may be specified for this mode.');
      | % elseif strcmp(mode, 'fields of arbitrary size')
      | %     current_names = textscan(strtrim(strrep(strrep(get_param(blk, 'names'), ']', ''), '[', '')), '%s');
      | %     current_names = current_names{1};
      | %     numios = length(current_names);
      | %     if length(current_widths) ~= numios,
      | %         error('%d field names specified, but %d widths?', numios, length(current_widths));
      | %     end
      | % end
      | % total_width = 0;
      | % for ctr = 1 : length(current_widths),
      | %     total_width = total_width + current_widths(ctr);
      | % end
      | % if total_width > 32,
      | %     error('Total width must be 32 or less, set to %d.', total_width);
      | % end
      mask Callback arith_types:
      | [numios, ~, ~, ~, current_types] = swreg_maskcheck(gcb);
      | % blk = gcb;
      | % mode = get_param(blk, 'mode');
      | % current_types = eval(get_param(blk, 'arith_types'));
      | % numios = length(current_types);
      | % if (strcmp(mode, 'one value') || strcmp(mode, 'fields of equal size')) && (length(current_types) > 1),
      | %     error('Only one type may be specified for this mode.');
      | % elseif strcmp(mode, 'fields of arbitrary size')
      | %     current_names = textscan(strtrim(strrep(strrep(get_param(blk, 'names'), ']', ''), '[', '')), '%s');
      | %     current_names = current_names{1};
      | %     numios = length(current_names);
      | %     if length(current_types) ~= numios,
      | %         error('%d field names specified, but %d types?', numios, length(current_types));
      | %     end
      | % end
      | problem = 0;
      | for ctr = 1 : numios,
      |     t = current_types(ctr);
      |     if (t < 0) || (t > 2),
      |         problem = t;
      |         ctr = numios + 1;
      |     end
      | end
      | if problem ~= 0,
      |     error('Type cannot be %i, must be 0, 1 or 2.', problem);
      | end
      mask Callback bin_pts:
      | swreg_maskcheck(gcb);
      | % blk = gcb;
      | % mode = get_param(blk, 'mode');
      | % current_bins = eval(get_param(blk, 'bin_pts'));
      | % if (strcmp(mode, 'one value') || strcmp(mode, 'fields of equal size')) && (length(current_bins) > 1),
      | %     error('Only one binary pt may be specified for this mode.');
      | % elseif strcmp(mode, 'fields of arbitrary size')
      | %     current_names = textscan(strtrim(strrep(strrep(get_param(blk, 'names'), ']', ''), '[', '')), '%s');
      | %     current_names = current_names{1};
      | %     numios = length(current_names);
      | %     if length(current_bins) ~= numios,
      | %         error('%d field names specified, but %d binary pts?', numios, length(current_bins));
      | %     end
      | % end
  Cos0 : Outport
  Cos1 : Outport  Port=2
  Cos2 : Outport  Port=3
  Cos3 : Outport  Port=4
  nSin0 : Outport  Port=5
  nSin1 : Outport  Port=6
  nSin2 : Outport  Port=7
  nSin3 : Outport  Port=8
  Buss : Outport  Port=9
  wires:
  Reinterpret4/1 -> Concat/5
  [cos2_] -> Mux2/4
  [sin0_] -> Mux5/2
  [cos0_] -> Mux4/2
  Constant6/1 -> sampleorder/1(sim_1)
  [sin1_] -> Mux5/3
  Reinterpret1/1 -> Concat/2
  Reinterpret/1 -> Concat/1
  [cos2_] -> Mux1/4
  bit_3_2_/1 -> [order1]
  Reinterpret3/1 -> Concat/4
  [cos0_] -> Mux3/2
  [cos1_] -> Mux4/3
  bit_7_6_/1 -> [order3]
  [cos0_] -> Mux1/2
  Mux7/1 -> nSin1/1, Reinterpret5/1
  Mux1/1 -> Reinterpret/1, Cos0/1
  Mux8/1 -> nSin0/1, Reinterpret4/1
  Reinterpret5/1 -> Concat/6
  [sin2_] -> Mux5/4
  Mux4/1 -> Cos3/1, Reinterpret3/1
  [cos1_] -> Mux1/3
  Reinterpret6/1 -> Concat/7
  [order3] -> Mux5/1
  Concat/1 -> Buss/1
  [cos3_] -> Mux1/5
  Mux2/1 -> Cos1/1, Reinterpret1/1
  [cos2_] -> Mux4/4
  sampleorder/1(in_reg) -> bit_7_6_/1, bit_5_4_/1, bit_3_2_/1, bit_1_0_/1
  Mux5/1 -> nSin3/1, Reinterpret7/1
  [sin2_] -> Mux8/4
  [order1] -> Mux7/1
  [cos3_] -> Mux3/5
  [order1] -> Mux2/1
  [order2] -> Mux6/1
  i0/1 -> [cos0_]
  Mux6/1 -> nSin2/1, Reinterpret6/1
  [cos2_] -> Mux3/4
  [sin0_] -> Mux7/2
  [cos0_] -> Mux2/2
  [sin3_] -> Mux7/5
  [sin2_] -> Mux7/4
  [cos1_] -> Mux3/3
  [sin0_] -> Mux8/2
  [order0] -> Mux8/1
  [sin3_] -> Mux5/5
  bit_1_0_/1 -> [order0]
  [cos3_] -> Mux4/5
  [sin1_] -> Mux7/3
  [cos1_] -> Mux2/3
  [sin1_] -> Mux8/3
  [order3] -> Mux4/1
  [sin1_] -> Mux6/3
  Reinterpret7/1 -> Concat/8
  q3/1 -> [sin3_]
  [sin3_] -> Mux6/5
  Mux3/1 -> Cos2/1, Reinterpret2/1
  bit_5_4_/1 -> [order2]
  [sin3_] -> Mux8/5
  [sin2_] -> Mux6/4
  Reinterpret2/1 -> Concat/3
  [cos3_] -> Mux2/5
  [order0] -> Mux1/1
  [order2] -> Mux3/1
  [sin0_] -> Mux6/2
  q2/1 -> [sin2_]
  q1/1 -> [sin1_]
  q0/1 -> [sin0_]
  i3/1 -> [cos3_]
  i1/1 -> [cos1_]
  i2/1 -> [cos2_]

== system maddenlibrary/MKID_DAC/buss128toIQ1 ==
  In1 : Inport
  Reinterpret{1..8} (8 alike) : xbsIndex_r4/Reinterpret  force_arith_type=on  arith_type="Signed  (2's comp)"  force_bin_pt=on  bin_pt=15  block_type=reinterpret
      settings: infoedit="Changes signal type without altering the binary representation.   You can changed the signal between signed and unsigned, and relocate the binary point.<P><P>Hardware notes: In hardware this block costs nothing.<P><P>Example:  Suppose the input is 6 bits wide, signed, with 2 fractional bits, and the output is forced to unsigned with 0 fractional bits.  Then an input of -2.0 (1110.00 in binary 2's complement) becomes an output of 56 (111000 in binary)."  block_version=10.1.3
  data_111_96_ : xbsIndex_r4/Slice  nbits=16  boolean_output=off  mode=Lower Bit Location + Width  bit1=0  base1=LSB of Input  bit0=96  base0=LSB of Input  dbl_ovrd=off  block_type=slice
  data_127_112_ : xbsIndex_r4/Slice  nbits=16  boolean_output=off  mode=Lower Bit Location + Width  bit1=0  base1=LSB of Input  bit0=112  base0=LSB of Input  dbl_ovrd=off  block_type=slice
  data_15_0_ : xbsIndex_r4/Slice  nbits=16  boolean_output=off  mode=Lower Bit Location + Width  bit1=0  base1=LSB of Input  bit0=0  base0=LSB of Input  dbl_ovrd=off  block_type=slice
  data_31_16_ : xbsIndex_r4/Slice  nbits=16  boolean_output=off  mode=Lower Bit Location + Width  bit1=0  base1=LSB of Input  bit0=16  base0=LSB of Input  dbl_ovrd=off  block_type=slice
  data_47_32_ : xbsIndex_r4/Slice  nbits=16  boolean_output=off  mode=Lower Bit Location + Width  bit1=0  base1=LSB of Input  bit0=32  base0=LSB of Input  dbl_ovrd=off  block_type=slice
  data_63_48_ : xbsIndex_r4/Slice  nbits=16  boolean_output=off  mode=Lower Bit Location + Width  bit1=0  base1=LSB of Input  bit0=48  base0=LSB of Input  dbl_ovrd=off  block_type=slice
  data_79_64_ : xbsIndex_r4/Slice  nbits=16  boolean_output=off  mode=Lower Bit Location + Width  bit1=0  base1=LSB of Input  bit0=64  base0=LSB of Input  dbl_ovrd=off  block_type=slice
  data_95_80_ : xbsIndex_r4/Slice  nbits=16  boolean_output=off  mode=Lower Bit Location + Width  bit1=0  base1=LSB of Input  bit0=80  base0=LSB of Input  dbl_ovrd=off  block_type=slice
  I0 : Outport
  I1 : Outport  Port=2
  I2 : Outport  Port=3
  I3 : Outport  Port=4
  Q0 : Outport  Port=5
  Q1 : Outport  Port=6
  Q2 : Outport  Port=7
  Q3 : Outport  Port=8
  wires:
  Reinterpret1/1 -> I1/1
  Reinterpret5/1 -> Q1/1
  Reinterpret7/1 -> Q3/1
  data_111_96_/1 -> Reinterpret6/1
  Reinterpret6/1 -> Q2/1
  Reinterpret3/1 -> I3/1
  Reinterpret8/1 -> Q0/1
  data_63_48_/1 -> Reinterpret3/1
  data_31_16_/1 -> Reinterpret1/1
  data_79_64_/1 -> Reinterpret8/1
  data_47_32_/1 -> Reinterpret2/1
  data_95_80_/1 -> Reinterpret5/1
  In1/1 -> data_127_112_/1, data_111_96_/1, data_95_80_/1, data_79_64_/1, data_63_48_/1, data_47_32_/1, data_31_16_/1, data_15_0_/1
  data_15_0_/1 -> Reinterpret4/1
  data_127_112_/1 -> Reinterpret7/1
  Reinterpret4/1 -> I0/1
  Reinterpret2/1 -> I2/1

== system maddenlibrary/MKID_DAC/config ==
  sim_1 : Inport
  qdrdac_MKID_DAC_config_user_data_out : xbsIndex_r4/Gateway In  gui_display_data_type=Fixed-point  arith_type=Unsigned  n_bits=32  bin_pt=0  preci_type=Single  exp_width=8  frac_width=24  quantization="Round  (unbiased: +/- Inf)"  overflow=Saturate  period=1  dbl_ovrd=off  timing_constraint=None  locs_specified=off  LOCs={}  UseAsADC=off  ADCChannel='1'  inherit_from_input=off  hdl_port=on  block_type=gatewayin
  reint1 : xbsIndex_r4/Reinterpret  force_arith_type=on  arith_type=Unsigned  force_bin_pt=on  bin_pt=0  block_type=reinterpret
  slice_reg : xbsIndex_r4/Slice  nbits=32  boolean_output=off  mode=Lower Bit Location + Width  bit1=0  base1=MSB of Input  bit0=0  base0=LSB of Input  dbl_ovrd=off  block_type=slice
  in_reg : Outport
  wires:
  qdrdac_MKID_DAC_config_user_data_out/1 -> ?
  sim_1/1 -> qdrdac_MKID_DAC_config_user_data_out/1
  ? -> slice_reg/1
  slice_reg/1 -> reint1/1
  reint1/1 -> in_reg/1
